simulink model "EKFsim"  (R2024b)
settings: Solver=VariableStepAuto  StartTime=0.0  StopTime=param.simul.t_end  FixedStep=1/52  RelTol=1e-3
values from neighbouring files (symbols this model uses):
  N = length(t)    [trajectory_paraglider.m]    (also in trajectory_paraglider.mat = 31201; trajectory_paraglider_backup.m; unit_test_madgwick_full_traj.m)
undefined symbols (not defined in the file or in its folder): param
libraries: nesl_utility x7, sm_lib x4
settings Model: Creator=OBWELUC  LastModifiedBy=OBWELUC
settings ExplorerConfigSet: InternalSimMechanicsExplorerSettings="<ExplorerConfiguration><canonicalview>default</canonicalview><AnimationSetting><BasePlaybackSpeed>1.0</BasePlaybackSpeed><PlaybackSpeedFactor>0.00390625</PlaybackSpeedFactor></AnimationSetting><TilePanel><TileInfo><Tiles Columns=\"2\" Count=\"4\" Rows=\"2\"><Column Weight=\"0.4997\"/><Column Weight=\"0.5003\"/><Row Weight=\"0.5\"/><Row Weight=\"0.5\"/><Tile Height=\"1\" Width=\"1\" X=\"0\" Y=\"0\"/><Tile Height=\"1\" Width=\"1\" X=\"0\" Y=\"1\"/><Tile Height=\"1\" Width=\"1\" X=\"1\" Y=\"0\"/><Tile Height=\"1\" Width=\"1\" X=\"1\" Y=\"1\"/></Tiles></TileInfo><SceneInfo><SceneViewer><BGColor><R>0.60000002384185791</R><G>0.60000002384185791</G><B>0.60000002384185791</B></BGColor><Camera><DoPerspective>off</DoPerspective><Position><X>5.29153282342771369</X><Y>-4.80631047053996685</Y><Z>2.23047224175609227</Z></Position><Center><X>1.33679013155167015</X><Y>-8.50343425895516702e-07</Y><Z>1.79372941692059129</Z></Center><Up><X>-0.00245210583782279334</X><Y>0.0884942118943543576</Y><Z>0.996073672796424003</Z></Up><ViewLimDist>1</ViewLimDist><YLim>3.61698657274246216</YLim><XLim>5.76316532752325905</XLim></Camera></SceneViewer><SceneViewer><BGColor><R>0.60000002384185791</R><G>0.60000002384185791</G><B>0.60000002384185791</B></BGColor><Camera><DoPerspective>off</DoPerspective><Position><X>2.82812637171379455</X><Y>-3.86128984680013376</Y><Z>6.51831083835967462</Z></Position><Center><X>1.10088169185850537</X><Y>-0.0853434819935348088</Y><Z>2.80557330046554076</Z></Center><Up><X>0.0701428928981585736</X><Y>0.715516230746083615</Y><Z>0.695065822864852967</Z></Up><ViewLimDist>1</ViewLimDist><YLim>5.65757834911346436</YLim><XLim>9.01456467244634929</XLim></Camera></SceneViewer><SceneViewer><BGColor><R>0.60000002384185791</R><G>0.60000002384185791</G><B>0.60000002384185791</B></BGColor><Camera><DoPerspective>off</DoPerspective><Position><X>7.61755312712227983</X><Y>-8.51291863668279802e-08</Y><Z>1.79376937141421422</Z></Position><Center><X>1.33679044539985625</X><Y>-8.51291863668279802e-08</Y><Z>1.79376937141421422</Z></Center><Up><X>-0</X><Y>0</Y><Z>1</Z></Up><ViewLimDist>1</ViewLimDist><YLim>3.61698657274246216</YLim><XLim>5.77066944904347245</XLim></Camera></SceneViewer><SceneViewer><BGColor><R>0.60000002384185791</R><G>0.60000002384185791</G><B>0.60000002384185791</B></BGColor><Camera><DoPerspective>off</DoPerspective><Position><X>4.61649383527782309</X><Y>-3.27970335927912426</Y><Z>6.03338553158868862</Z></Position><Center><X>1.39001899753018088</X><Y>-0.0532285215318148985</Y><Z>2.80691069384086322</Z></Center><Up><X>-0.408248290463863073</X><Y>0.408248290463863073</Y><Z>0.816496580927726145</Z></Up><ViewLimDist>1</ViewLimDist><YLim>4.68673889160156243</YLim><XLim>7.4773904722854807</XLim></Camera></SceneViewer></SceneInfo></TilePanel><MechEditorPanel><Cameras/><GfxPanelCameraMap/><VideoCreator><PlaybackSpeedRatio>1.0</PlaybackSpeedRatio><FrameRate>30</FrameRate><VideoFormat>Motion JPEG AVI</VideoFormat><FrameSize>auto</FrameSize></VideoCreator></MechEditorPanel></ExplorerConfiguration>"

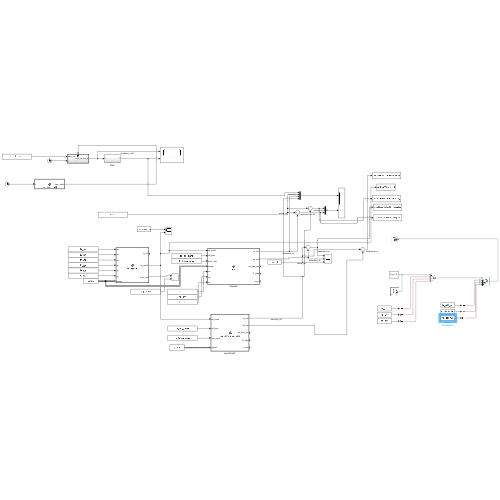
[thumbnail: Simulink's stored preview of the top-level diagram]
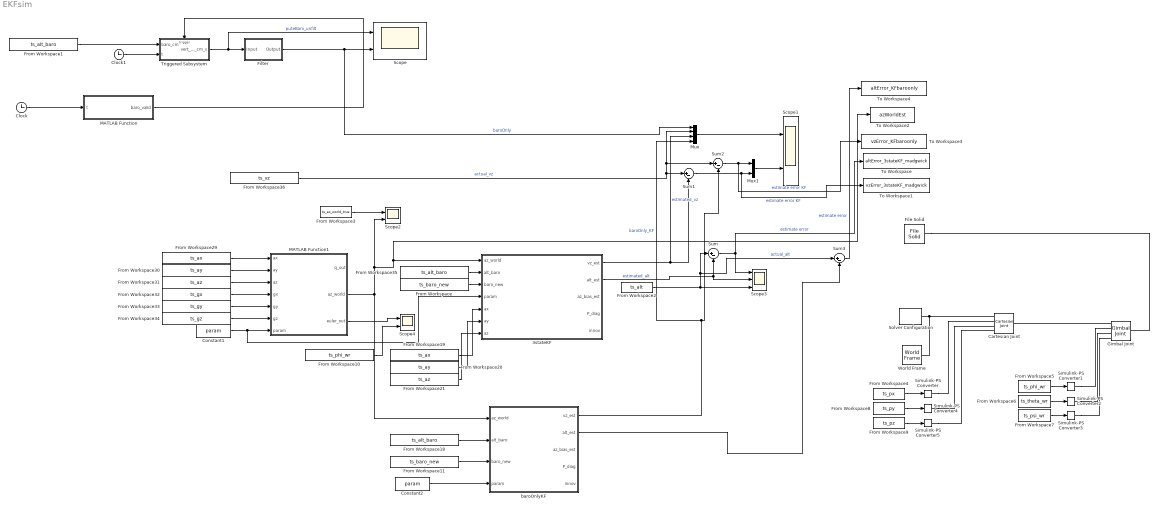
== system EKFsim ==
  3stateKF : MATLAB Function  TreatAsAtomicUnit=on  SystemSampleTime=param.dt_imu
  Cartesian Joint : sm_lib/Joints/Cartesian Joint  JointMode=Normal  CompositeWrenchDir=FollowerOnBase  CompositeWrenchFrame=BaseFrame  SenseConstraintForce=off  SenseConstraintTorque=off  SenseTotalForce=off  SenseTotalTorque=off  PxPositionTargetSpecify=off  PxPositionTargetPriority=High  PxPositionTargetValue=0  PxPositionTargetValueUnits=m  PxVelocityTargetSpecify=off  PxVelocityTargetPriority=High  PxVelocityTargetValue=0  PxVelocityTargetValueUnits=m/s  PxEquilibriumPosition=0  PxEquilibriumPositionUnits=m  PxSpringStiffness=0  PxSpringStiffnessUnits=N/m  PxDampingCoefficient=0  PxDampingCoefficientUnits=N/(m/s)  PxLowerLimitSpecify=off  PxLowerLimitBound=-1  PxLowerLimitBoundUnits=m  PxLowerLimitStiffness=1e6  PxLowerLimitStiffnessUnits=N/m  PxLowerLimitDamping=1e3  PxLowerLimitDampingUnits=N/(m/s)  PxLowerLimitTransitionRegionWidth=1e-4  PxLowerLimitTransitionRegionWidthUnits=m  PxUpperLimitSpecify=off  PxUpperLimitBound=1  PxUpperLimitBoundUnits=m  PxUpperLimitStiffness=1e6  PxUpperLimitStiffnessUnits=N/m  PxUpperLimitDamping=1e3  PxUpperLimitDampingUnits=N/(m/s)  PxUpperLimitTransitionRegionWidth=1e-4  PxUpperLimitTransitionRegionWidthUnits=m  PxTorqueActuationMode=ComputedTorque  PxMotionActuationMode=InputMotion  PxSensePosition=off  PxSenseVelocity=off  PxSenseAcceleration=off  PxSenseTorqueForce=off  PxSenseLowerLimitTorqueForce=off  PxSenseUpperLimitTorqueForce=off  PyPositionTargetSpecify=off  PyPositionTargetPriority=High  PyPositionTargetValue=0  PyPositionTargetValueUnits=m  PyVelocityTargetSpecify=off  PyVelocityTargetPriority=High  PyVelocityTargetValue=0  PyVelocityTargetValueUnits=m/s  PyEquilibriumPosition=0  PyEquilibriumPositionUnits=m  PySpringStiffness=0  PySpringStiffnessUnits=N/m  PyDampingCoefficient=0  PyDampingCoefficientUnits=N/(m/s)  PyLowerLimitSpecify=off  PyLowerLimitBound=-1  PyLowerLimitBoundUnits=m  PyLowerLimitStiffness=1e6  PyLowerLimitStiffnessUnits=N/m  PyLowerLimitDamping=1e3  PyLowerLimitDampingUnits=N/(m/s)  PyLowerLimitTransitionRegionWidth=1e-4  PyLowerLimitTransitionRegionWidthUnits=m  PyUpperLimitSpecify=off  PyUpperLimitBound=1  PyUpperLimitBoundUnits=m  PyUpperLimitStiffness=1e6  PyUpperLimitStiffnessUnits=N/m  PyUpperLimitDamping=1e3  PyUpperLimitDampingUnits=N/(m/s)  PyUpperLimitTransitionRegionWidth=1e-4  PyUpperLimitTransitionRegionWidthUnits=m  PyTorqueActuationMode=ComputedTorque  PyMotionActuationMode=InputMotion  PySensePosition=off  PySenseVelocity=off  PySenseAcceleration=off  PySenseTorqueForce=off  PySenseLowerLimitTorqueForce=off  PySenseUpperLimitTorqueForce=off  PzPositionTargetSpecify=off  PzPositionTargetPriority=High  PzPositionTargetValue=0  PzPositionTargetValueUnits=m  PzVelocityTargetSpecify=off  PzVelocityTargetPriority=High  PzVelocityTargetValue=0  PzVelocityTargetValueUnits=m/s  PzEquilibriumPosition=0  PzEquilibriumPositionUnits=m  PzSpringStiffness=0  PzSpringStiffnessUnits=N/m  PzDampingCoefficient=0  PzDampingCoefficientUnits=N/(m/s)  PzLowerLimitSpecify=off  PzLowerLimitBound=-1  PzLowerLimitBoundUnits=m  PzLowerLimitStiffness=1e6  PzLowerLimitStiffnessUnits=N/m  PzLowerLimitDamping=1e3  PzLowerLimitDampingUnits=N/(m/s)  PzLowerLimitTransitionRegionWidth=1e-4  PzLowerLimitTransitionRegionWidthUnits=m  PzUpperLimitSpecify=off  PzUpperLimitBound=1  PzUpperLimitBoundUnits=m  PzUpperLimitStiffness=1e6  PzUpperLimitStiffnessUnits=N/m  PzUpperLimitDamping=1e3  PzUpperLimitDampingUnits=N/(m/s)  PzUpperLimitTransitionRegionWidth=1e-4  PzUpperLimitTransitionRegionWidthUnits=m  PzTorqueActuationMode=ComputedTorque  PzMotionActuationMode=InputMotion  PzSensePosition=off  PzSenseVelocity=off  PzSenseAcceleration=off  PzSenseTorqueForce=off  PzSenseLowerLimitTorqueForce=off  PzSenseUpperLimitTorqueForce=off
  Clock : Clock
  Clock1 : Clock
  Constant1 : Constant  Value=param  OutDataTypeStr=Bus: BusKF
  Constant2 : Constant  Value=param  OutDataTypeStr=Bus: BusKF
  File Solid : sm_lib/Body Elements/File Solid  ExtGeomFileName=C:\Users\OBWELUC\Desktop\miniVarioCode\kf\Assemblage paramoteur.STEP  UnitType=FromFile  ExtGeomFileUnits=m  StepReaderType=HEX  ExportConvexHullGeometry=off  InertiaType=PointMass  BasedOnType=DensityFromFile  Density=1000  DensityUnits=kg/m^3  Mass=1  MassUnits=kg  CenterOfMass=[0 0 0]  CenterOfMassUnits=m  MomentsOfInertia=[1 1 1]  MomentsOfInertiaUnits=kg*m^2  ProductsOfInertia=[0 0 0]  ProductsOfInertiaUnits=kg*m^2  GraphicType=FromGeometry  MarkerShape=Sphere  MarkerSize=10  GraphicVisPropType=SimpleVisualProperties  GraphicDiffuseColor=[0.5 0.5 0.5]  GraphicOpacity=1  GraphicSpecularColor=[0.5 0.5 0.5 1.0]  GraphicAmbientColor=[0.15 0.15 0.15 1.0]  GraphicEmissiveColor=[0.0 0.0 0.0 1.0]  GraphicShininess=75  DoExposeReferenceFrame=off  SerializedFrames=<Frames><Frame><Id>Frame1</Id><Value><Name>Fcorr</Name><Origin><Source>ReferenceFrame</Source><FeatureName></FeatureName></Origin><PrimaryAxis><DefinedDirection>+X</DefinedDirection><Source>ReferenceFrame</Source><SourceDirection>+Z</SourceDirection><FeatureName></FeatureName></PrimaryAxis><SecondaryAxis><DefinedDirection>+Y</DefinedDirection><Source>ReferenceFrame</Source><SourceDirection>+X</SourceDirection><FeatureName></FeatureName></SecondaryAxis></Value></Frame></Frames>
  Filter : Subsystem  Tag=FilterWizardSubSystem
      settings: ErrorFcn=dspFilterRealizedInBasicElemsAlgLoopErrFcnCallback
  From Workspace : FromWorkspace  VariableName=ts_baro_new  SampleTime=param.dt_imu
  From Workspace1 : FromWorkspace  VariableName=ts_alt_baro  SampleTime=1/52
  From Workspace10 : FromWorkspace  VariableName=ts_phi_wr  SampleTime=param.dt_imu
  From Workspace11 : FromWorkspace  VariableName=ts_baro_new  SampleTime=param.dt_imu
  From Workspace18 : FromWorkspace  VariableName=ts_alt_baro  SampleTime=param.dt_imu
  From Workspace19 : FromWorkspace  VariableName=ts_ax  SampleTime=param.dt_imu
  From Workspace2 : FromWorkspace  VariableName=ts_alt  SampleTime=1/52
  From Workspace20 : FromWorkspace  VariableName=ts_ay  SampleTime=param.dt_imu
  From Workspace21 : FromWorkspace  VariableName=ts_az  SampleTime=param.dt_imu
  From Workspace29 : FromWorkspace  VariableName=ts_ax  SampleTime=param.dt_imu
  From Workspace3 : FromWorkspace  VariableName=ts_az_world_true
  From Workspace30 : FromWorkspace  VariableName=ts_ay  SampleTime=param.dt_imu
  From Workspace31 : FromWorkspace  VariableName=ts_az  SampleTime=param.dt_imu
  From Workspace32 : FromWorkspace  VariableName=ts_gx  SampleTime=param.dt_imu
  From Workspace33 : FromWorkspace  VariableName=ts_gy  SampleTime=param.dt_imu
  From Workspace34 : FromWorkspace  VariableName=ts_gz  SampleTime=param.dt_imu
  From Workspace35 : FromWorkspace  VariableName=ts_alt_baro  SampleTime=param.dt_imu
  From Workspace36 : FromWorkspace  VariableName=ts_vz  SampleTime=1/52
  From Workspace4 : FromWorkspace  VariableName=ts_px  SampleTime=-1
  From Workspace5 : FromWorkspace  VariableName=ts_phi_wr  SampleTime=-1
  From Workspace6 : FromWorkspace  VariableName=ts_theta_wr  SampleTime=-1
  From Workspace7 : FromWorkspace  VariableName=ts_psi_wr  SampleTime=-1
  From Workspace8 : FromWorkspace  VariableName=ts_py  SampleTime=-1
  From Workspace9 : FromWorkspace  VariableName=ts_pz  SampleTime=-1
  Gimbal Joint : sm_lib/Joints/Gimbal Joint  JointMode=Normal  CompositeWrenchDir=FollowerOnBase  CompositeWrenchFrame=BaseFrame  SenseConstraintForce=off  SenseConstraintTorque=off  SenseTotalForce=off  SenseTotalTorque=off  RxPositionTargetSpecify=off  RxPositionTargetPriority=High  RxPositionTargetValue=0  RxPositionTargetValueUnits=deg  RxVelocityTargetSpecify=off  RxVelocityTargetPriority=High  RxVelocityTargetValue=0  RxVelocityTargetValueUnits=deg/s  RxEquilibriumPosition=0  RxEquilibriumPositionUnits=deg  RxSpringStiffness=0  RxSpringStiffnessUnits=N*m/deg  RxDampingCoefficient=0  RxDampingCoefficientUnits=N*m/(deg/s)  RxLowerLimitSpecify=off  RxLowerLimitBound=-90  RxLowerLimitBoundUnits=deg  RxLowerLimitStiffness=1e4  RxLowerLimitStiffnessUnits=N*m/deg  RxLowerLimitDamping=10  RxLowerLimitDampingUnits=N*m/(deg/s)  RxLowerLimitTransitionRegionWidth=0.1  RxLowerLimitTransitionRegionWidthUnits=deg  RxUpperLimitSpecify=off  RxUpperLimitBound=90  RxUpperLimitBoundUnits=deg  RxUpperLimitStiffness=1e4  RxUpperLimitStiffnessUnits=N*m/deg  RxUpperLimitDamping=10  RxUpperLimitDampingUnits=N*m/(deg/s)  RxUpperLimitTransitionRegionWidth=0.1  RxUpperLimitTransitionRegionWidthUnits=deg  RxTorqueActuationMode=ComputedTorque  RxMotionActuationMode=InputMotion  RxSensePosition=off  RxSenseVelocity=off  RxSenseAcceleration=off  RxSenseTorqueForce=off  RxSenseLowerLimitTorqueForce=off  RxSenseUpperLimitTorqueForce=off  RyPositionTargetSpecify=off  RyPositionTargetPriority=High  RyPositionTargetValue=0  RyPositionTargetValueUnits=deg  RyVelocityTargetSpecify=off  RyVelocityTargetPriority=High  RyVelocityTargetValue=0  RyVelocityTargetValueUnits=deg/s  RyEquilibriumPosition=0  RyEquilibriumPositionUnits=deg  RySpringStiffness=0  RySpringStiffnessUnits=N*m/deg  RyDampingCoefficient=0  RyDampingCoefficientUnits=N*m/(deg/s)  RyLowerLimitSpecify=off  RyLowerLimitBound=-90  RyLowerLimitBoundUnits=deg  RyLowerLimitStiffness=1e4  RyLowerLimitStiffnessUnits=N*m/deg  RyLowerLimitDamping=10  RyLowerLimitDampingUnits=N*m/(deg/s)  RyLowerLimitTransitionRegionWidth=0.1  RyLowerLimitTransitionRegionWidthUnits=deg  RyUpperLimitSpecify=off  RyUpperLimitBound=90  RyUpperLimitBoundUnits=deg  RyUpperLimitStiffness=1e4  RyUpperLimitStiffnessUnits=N*m/deg  RyUpperLimitDamping=10  RyUpperLimitDampingUnits=N*m/(deg/s)  RyUpperLimitTransitionRegionWidth=0.1  RyUpperLimitTransitionRegionWidthUnits=deg  RyTorqueActuationMode=ComputedTorque  RyMotionActuationMode=InputMotion  RySensePosition=off  RySenseVelocity=off  RySenseAcceleration=off  RySenseTorqueForce=off  RySenseLowerLimitTorqueForce=off  RySenseUpperLimitTorqueForce=off  RzPositionTargetSpecify=off  RzPositionTargetPriority=High  RzPositionTargetValue=0  RzPositionTargetValueUnits=deg  RzVelocityTargetSpecify=off  RzVelocityTargetPriority=High  RzVelocityTargetValue=0  RzVelocityTargetValueUnits=deg/s  RzEquilibriumPosition=0  RzEquilibriumPositionUnits=deg  RzSpringStiffness=0  RzSpringStiffnessUnits=N*m/deg  RzDampingCoefficient=0  RzDampingCoefficientUnits=N*m/(deg/s)  RzLowerLimitSpecify=off  RzLowerLimitBound=-90  RzLowerLimitBoundUnits=deg  RzLowerLimitStiffness=1e4  RzLowerLimitStiffnessUnits=N*m/deg  RzLowerLimitDamping=10  RzLowerLimitDampingUnits=N*m/(deg/s)  RzLowerLimitTransitionRegionWidth=0.1  RzLowerLimitTransitionRegionWidthUnits=deg  RzUpperLimitSpecify=off  RzUpperLimitBound=90  RzUpperLimitBoundUnits=deg  RzUpperLimitStiffness=1e4  RzUpperLimitStiffnessUnits=N*m/deg  RzUpperLimitDamping=10  RzUpperLimitDampingUnits=N*m/(deg/s)  RzUpperLimitTransitionRegionWidth=0.1  RzUpperLimitTransitionRegionWidthUnits=deg  RzTorqueActuationMode=ComputedTorque  RzMotionActuationMode=InputMotion  RzSensePosition=off  RzSenseVelocity=off  RzSenseAcceleration=off  RzSenseTorqueForce=off  RzSenseLowerLimitTorqueForce=off  RzSenseUpperLimitTorqueForce=off
  MATLAB Function : MATLAB Function  TreatAsAtomicUnit=on
  MATLAB Function1 : MATLAB Function  TreatAsAtomicUnit=on  SystemSampleTime=param.dt_imu
  Mux : Mux
  Mux1 : Mux  Inputs=2
  Scope{,1..2,4} (4 alike) : Scope  NumInputPorts=2
  Scope3 : Scope  NumInputPorts=3
  Simulink-PS Converter{,1..5} (6 alike) : nesl_utility/Simulink-PS Converter  PhysicalDomain=network_engine_domain  SubClassName=ps_input  LeftPortType=input  RightPortType=output  PseudoPeriodic=off  Frequencies=[]  NoiseDistribution=none  NoiseParameters=[]  Unit=1  AffineConversion=off  FilteringAndDerivatives=filter  SimscapeFilterOrder=2  InputFilterTimeConstant=0.001  UdotUserProvided=0
  Solver Configuration : nesl_utility/Solver Configuration  PhysicalDomain=network_engine_domain  SubClassName=solver  LeftPortType=input  RightPortType=generic  Tones=[]  Harmonics=[]  SimulateNoise=off  Profile=off  UseLocalSampling=off  EnableSwitchedLinearOptims=on  FrequencyDomain=off  UseCCode=off  RelTol=0.001  AbsTol=0.001  MinStep=1e-09  ToWorkspace=off  RevertToSquareIcSolve=off  NumHomotopyIterations=100  PhasorMode=off  PhasorModeNumHarmonics=1  ConsistencySolver=NEWTON_XTOL_AFTER_FTOL  IndexReductionMethod=DerivativeReplacement  DoDC=off  ResidualTolerance=1e-09  ConsistencyTolSource=GLOBAL  ConsistencyAbsTol=0.001  ConsistencyRelTol=0.001  ConsistencyTolFactor=0.001  UseLocalSolver=off  LocalSolverChoice=NE_BACKWARD_EULER_ADVANCER  ResolveIndetEquations=on  FunctionEvalNumThread=1  LocalSolverSampleTime=0.001  DoFixedCost=off  MaxNonlinIter=3  MaxModeIter=2  ComputeImpulses=off  ImpulseIterations=2  LinearAlgebra=auto  LinearAlgebraNumThread=0  EquationFormulation=NE_TIME_EF  DelaysMemoryBudget=1024  AutomaticFiltering=on  FilteringTimeConstant=0.001  PartitionStorageMethod=AS_NEEDED  PartitionMemoryBudget=1024  PartitionMethod=ROBUST  MultibodyUseLocalSolver=off  MultibodyLocalSolverChoice=ODE1  MultibodyLocalSolverSampleTime=0.001
  Sum{,1..3} (4 alike) : Sum  Inputs=|+-
  To Workspace : ToWorkspace  VariableName=altError_3stateKF_madgwick  SaveFormat=Timeseries  SampleTime=-1
  To Workspace1 : ToWorkspace  VariableName=vzError_3stateKF_madgwick  SaveFormat=Timeseries  SampleTime=-1
  To Workspace2 : ToWorkspace  VariableName=azWorldEst  SaveFormat=Timeseries  SampleTime=-1
  To Workspace3 : ToWorkspace  VariableName=vzError_KFbaroonly  SaveFormat=Timeseries  SampleTime=-1
  To Workspace4 : ToWorkspace  VariableName=altError_KFbaroonly  SaveFormat=Timeseries  SampleTime=-1
  Triggered Subsystem : Subsystem  TreatAsAtomicUnit=on
  World Frame : sm_lib/Frames and Transforms/World Frame
  baroOnlyKF : MATLAB Function  TreatAsAtomicUnit=on
  wires:
  MATLAB Function/1(baro_valid) -> Triggered Subsystem/Trigger
  Clock/1 -> MATLAB Function/1(t)
  Clock1/1 -> Triggered Subsystem/2(t)
  Triggered Subsystem/1(vert_vel_cm_s) -> Scope/1, Filter/1(Input)  "puteBaro_unfilt"
  Constant1/1 -> 3stateKF/4(param), MATLAB Function1/7(param)
  From Workspace29/1 -> MATLAB Function1/1(ax)
  From Workspace30/1 -> MATLAB Function1/2(ay)
  From Workspace31/1 -> MATLAB Function1/3(az)
  From Workspace32/1 -> MATLAB Function1/4(gx)
  From Workspace33/1 -> MATLAB Function1/5(gy)
  From Workspace34/1 -> MATLAB Function1/6(gz)
  MATLAB Function1/2(az_world) -> baroOnlyKF/1(az_world), 3stateKF/1(az_world), To Workspace2/1, Scope2/2
  From Workspace35/1 -> 3stateKF/2(alt_baro)
  From Workspace1/1 -> Triggered Subsystem/1(baro_cm)
  From Workspace/1 -> 3stateKF/3(baro_new)
  From Workspace4/1 -> Simulink-PS Converter/1
  From Workspace5/1 -> Simulink-PS Converter1/1
  From Workspace7/1 -> Simulink-PS Converter3/1
  From Workspace6/1 -> Simulink-PS Converter2/1
  From Workspace8/1 -> Simulink-PS Converter4/1
  From Workspace9/1 -> Simulink-PS Converter5/1
  3stateKF/2(alt_est) -> Scope3/2, Sum/2  "estimated_alt"
  From Workspace2/1 -> Sum3/1, Sum/1, Scope3/3  "actual_alt"
  Sum/1 -> Scope3/1, To Workspace/1  "estimate error"
  3stateKF/1(vz_est) -> Sum1/2, Mux/3  "estimated_vz"
  From Workspace36/1 -> Sum1/1, Sum2/1, Mux/2  "actual_vz"
  Filter/1(Output) -> Mux/1, Scope/2  "baroOnly"
  Mux/1 -> Scope1/1
  Mux1/1 -> Scope1/2
  Sum1/1 -> To Workspace1/1, Mux1/2  "estimate error KF"
  Sum2/1 -> To Workspace3/1, Mux1/1  "estimate error KF"
  From Workspace11/1 -> baroOnlyKF/3(baro_new)
  From Workspace18/1 -> baroOnlyKF/2(alt_baro)
  Constant2/1 -> baroOnlyKF/4(param)
  From Workspace19/1 -> 3stateKF/5(ax)
  From Workspace20/1 -> 3stateKF/6(ay)
  From Workspace21/1 -> 3stateKF/7(az)
  baroOnlyKF/1(vz_est) -> Mux/4, Sum2/2  "baroOnly_KF"
  From Workspace3/1 -> Scope2/1
  MATLAB Function1/3(euler_out) -> Scope4/1
  From Workspace10/1 -> Scope4/2
  baroOnlyKF/2(alt_est) -> Sum3/2
  Sum3/1 -> To Workspace4/1  "estimate error"
  connections:
  Solver Configuration/RConn1 -- Cartesian Joint/LConn1 -- World Frame/RConn1
  File Solid/LConn1 -- Gimbal Joint/RConn1
  Gimbal Joint/LConn1 -- Cartesian Joint/RConn1
  Simulink-PS Converter/RConn1 -- Cartesian Joint/LConn2
  Simulink-PS Converter2/RConn1 -- Gimbal Joint/LConn3
  Simulink-PS Converter1/RConn1 -- Gimbal Joint/LConn2
  Simulink-PS Converter3/RConn1 -- Gimbal Joint/LConn4
  Simulink-PS Converter4/RConn1 -- Cartesian Joint/LConn3
  Simulink-PS Converter5/RConn1 -- Cartesian Joint/LConn4

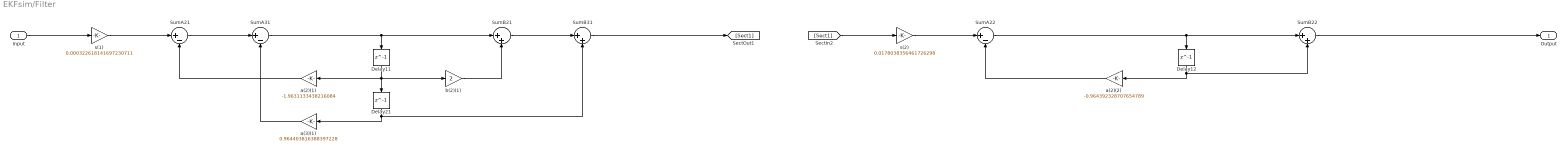
== system EKFsim/Filter ==
  Input : Inport
  Delay11 : Delay  DelayLength=1  InitialCondition=0
  Delay12 : Delay  DelayLength=1  InitialCondition=0
  Delay21 : Delay  DelayLength=1  InitialCondition=0
  SumA21 : Sum  Inputs=|+-  RndMeth=Nearest  SaturateOnIntegerOverflow=on  OutDataTypeStr=Inherit: Same as first input
  SumA22 : Sum  Inputs=|+-  RndMeth=Nearest  SaturateOnIntegerOverflow=on  OutDataTypeStr=Inherit: Same as first input
  SumA31 : Sum  Inputs=|+-  RndMeth=Nearest  SaturateOnIntegerOverflow=on  OutDataTypeStr=Inherit: Same as first input
  SumB21 : Sum  Inputs=|++  RndMeth=Nearest  SaturateOnIntegerOverflow=on  OutDataTypeStr=Inherit: Same as first input
  SumB22 : Sum  Inputs=|++  RndMeth=Nearest  SaturateOnIntegerOverflow=on  OutDataTypeStr=Inherit: Same as first input
  SumB31 : Sum  Inputs=|++  RndMeth=Nearest  SaturateOnIntegerOverflow=on  OutDataTypeStr=Inherit: Same as first input
  a(2)(1) : Gain  Gain=-1.9631133438216084  ParamDataTypeStr=double  RndMeth=Nearest  SaturateOnIntegerOverflow=on  OutDataTypeStr=Inherit: Same as input
  a(2)(2) : Gain  Gain=-0.964392328707654789  ParamDataTypeStr=double  RndMeth=Nearest  SaturateOnIntegerOverflow=on  OutDataTypeStr=Inherit: Same as input
  a(3)(1) : Gain  Gain=0.964403816388397228  ParamDataTypeStr=double  RndMeth=Nearest  SaturateOnIntegerOverflow=on  OutDataTypeStr=Inherit: Same as input
  b(2)(1) : Gain  Gain=2  ParamDataTypeStr=double  RndMeth=Nearest  SaturateOnIntegerOverflow=on  OutDataTypeStr=Inherit: Same as input
  s(1) : Gain  Gain=0.000322618141697230711  ParamDataTypeStr=double  RndMeth=Nearest  SaturateOnIntegerOverflow=on  OutDataTypeStr=Inherit: Same as input
  s(2) : Gain  Gain=0.0178038356461726298  ParamDataTypeStr=double  RndMeth=Nearest  SaturateOnIntegerOverflow=on  OutDataTypeStr=Inherit: Same as input
  Output : Outport
  wires:
  Input/1 -> s(1)/1
  s(1)/1 -> SumA21/1
  SumA21/1 -> SumA31/1
  SumA31/1 -> SumB21/1, Delay11/1
  SumB21/1 -> SumB31/1
  SumB31/1 -> [Sect1]
  a(2)(1)/1 -> SumA21/2
  Delay11/1 -> a(2)(1)/1, b(2)(1)/1, Delay21/1
  b(2)(1)/1 -> SumB21/2
  a(3)(1)/1 -> SumA31/2
  Delay21/1 -> a(3)(1)/1, SumB31/2
  [Sect1] -> s(2)/1
  s(2)/1 -> SumA22/1
  SumA22/1 -> SumB22/1, Delay12/1
  SumB22/1 -> Output/1
  a(2)(2)/1 -> SumA22/2
  Delay12/1 -> a(2)(2)/1, SumB22/2

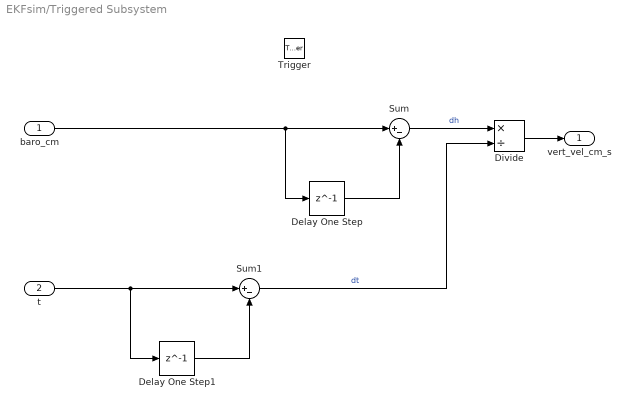
== system EKFsim/Triggered Subsystem ==
  baro_cm : Inport
  t : Inport  Port=2
  Trigger : TriggerPort  VariantControl=(inherit)
  Delay One Step : Delay  DelayLength=1
  Delay One Step1 : Delay  DelayLength=1
  Divide : Product  Inputs=*/
  Sum : Sum  Inputs=|+-
  Sum1 : Sum  Inputs=|+-
  vert_vel_cm_s : Outport
  wires:
  baro_cm/1 -> Sum/1, Delay One Step/1
  Delay One Step/1 -> Sum/2
  Sum/1 -> Divide/1  "dh"
  t/1 -> Delay One Step1/1, Sum1/1
  Delay One Step1/1 -> Sum1/2
  Sum1/1 -> Divide/2  "dt"
  Divide/1 -> vert_vel_cm_s/1

== matlab function EKFsim/MATLAB Function ==
  data: t input; baro_valid output
function baro_valid = gen_baro_valid(t)
  baro_valid = mod(round(t * 52), 7) == 0;
end

== matlab function EKFsim/3stateKF ==
  data: az_world input; vz_est output; alt_baro input; baro_new input; param input Bus: BusKF; alt_est output; az_bias_est output; P_diag output; innov output; ax input; ay input; az input
function [vz_est, alt_est, az_bias_est, P_diag, innov] = ...
         KF(az_world, alt_baro, baro_new, param, ax, ay, az)
    [vz_est, alt_est, az_bias_est, P_diag, innov] = fcn_kalman_vz(az_world, alt_baro, baro_new, param, ax, ay, az);
end

== matlab function EKFsim/MATLAB Function1 ==
  data: ax input; q_out output; ay input; az input; gx input; gy input; gz input; param input Bus: BusKF; az_world output; euler_out output
function [q_out, az_world, euler_out] = madgwick(ax, ay, az, gx, gy, gz, param)
    [q_out, az_world, euler_out] = fcn_madgwick(ax, ay, az, gx, gy, gz, param);
end

== matlab function EKFsim/baroOnlyKF ==
  data: az_world input; vz_est output; alt_baro input; baro_new input; param input Bus: BusKF; alt_est output; az_bias_est output; P_diag output; innov output
function [vz_est, alt_est, az_bias_est, P_diag, innov] = ...
         fcn_kalman_vz_baro(az_world, alt_baro, baro_new, param)
%FCN_KALMAN_VZ_BARO  Baro-primary Kalman filter for vertical speed estimation.
%
%  Architecture: barometer is the PRIMARY sensor and drives all meaningful
%  state corrections. The IMU (az_world from Madgwick) is used ONLY as a
%  predictor between baro samples — its contribution is heavily discounted
%  so that attitude errors during banked thermals do not corrupt the estimate.
%
%  Motivation: during banked turns (45°–55°), Madgwick's az_world contains
%  systematic tilt errors that are larger than the baro noise. Letting the
%  KF trust the IMU in those conditions actively worsens vz accuracy.
%  By setting u=0 (zero-acceleration prediction) and inflating Q to cover
%  the real vz dynamics, the baro update at 8 Hz carries the estimate and
%  the IMU error is absorbed into the process noise.
%
% =========================================================================
%  STATE VECTOR   x = [h; vz; az_bias]
%    h        : altitude above reference [m], up positive
%    vz       : vertical speed [m/s], up positive
%    az_bias  : residual vertical accel bias [m/s²] — kept for interface
%               compatibility; with u=0 it absorbs mean IMU offset.
%
%  INPUTS
%    az_world  : Madgwick world-frame vertical specific force [m/s²]
%                Used only when IMU blending is enabled (see IMU_BLEND_WEIGHT).
%                Set IMU_BLEND_WEIGHT=0 to ignore entirely.
%    alt_baro  : barometer altitude measurement [m]  (ZOH from 8 Hz)
%    baro_new  : flag — 1 = new baro sample this step, 0 = old
%    param     : parameter bus (param_init.m)
%
%  OUTPUTS  (identical interface to fcn_kalman_vz.m for drop-in replacement)
%    vz_est      : estimated vertical speed [m/s], up positive
%    alt_est     : estimated altitude [m]
%    az_bias_est : estimated accel bias [m/s²]
%    P_diag      : diagonal of P (3×1)
%    innov       : baro innovation [m]  (NaN when no new measurement)
%
%  KEY DESIGN CHOICES vs fcn_kalman_vz.m
%  -----------------------------------------------------------------------
%  1. Control input u = IMU_BLEND_WEIGHT * (-(az_world+g))
%     Default IMU_BLEND_WEIGHT = 0  →  zero-input prediction.
%     The predictor becomes: h_{k+1} = h_k + dt*vz_k
%                            vz_{k+1} = vz_k
%     vz is held constant between baro updates, which is correct on average
%     for a variometer (vz changes slowly relative to baro rate).
%
%  2. Q is set independently of param.kf.Q.
%     Q must be large enough that P grows sufficiently between baro updates
%     so the baro gain K is meaningful (~0.5–0.9 on the h channel).
%     Q_vz drives how quickly the filter can track vz changes.
%     Rule of thumb: sqrt(Q_vz * dt_baro) ≈ expected vz change per baro step.
%     At 8 Hz, a thermal onset can change vz by ~0.5 m/s in 0.125 s →
%     Q_vz ≈ (0.5/0.125)^2 * dt_imu ≈ 16 * (1/52) ≈ 0.31 m/s² per root-Hz.
%     We use a slightly more conservative value tunable via Q_VZ_SIGMA below.
%
%  3. Baro update uses the same R as param.kf.R_h (tunable separately).
%     The innovation gate is retained for outlier rejection.
%
%  SIMULINK USAGE
%    Drop-in replacement for fcn_kalman_vz.m.
%    Same port order, same sample time (param.dt_imu).
%    az_world input can be left connected — it is weighted to zero by default.
%
%#codegen

%% =========================================================
%  TUNING CONSTANTS  (edit here, not in param_init for now)
% ==========================================================

% Weight on IMU control input [0 = baro-only, 1 = full IMU trust]
% Set to 0 for pure baro-primary. Set to 0.1–0.3 to blend lightly.
IMU_BLEND_WEIGHT = 0;

% Process noise for vz [m/s per sqrt(Hz)]
% Governs how fast the filter tracks vz changes between baro updates.
% Increase if vz RMSE is large during rapid thermal entries.
% Decrease if the estimate is noisy during stable glide.
% Suggested range: 0.1 – 0.5
Q_VZ_SIGMA = 0.5;   % [m/s / sqrt(Hz)]

% Process noise for altitude [m per sqrt(Hz)]
% Usually much smaller than vz — altitude is the integrated state.
Q_H_SIGMA  = 0.01;  % [m / sqrt(Hz)]

% Process noise for bias [m/s² per sqrt(Hz)]
% With u=0, the bias state absorbs the mean IMU offset.
% Keep small so it doesn't destabilise; it's largely irrelevant here.
Q_BIAS_SIGMA = 0.005;  % [m/s² / sqrt(Hz)]

%% =========================================================
%  PERSISTENT STATE
% ==========================================================
persistent x_est P initialised;

if isempty(initialised)
    x_est      = param.kf.x0(:);
    x_est(1)   = alt_baro;        % warm-start altitude from first baro reading
    P          = param.kf.P0;
    initialised = true;
end

%% =========================================================
%  SYSTEM MATRICES
% ==========================================================
g    = param.simul.g;
dt   = param.dt_imu;

% State transition — identical to original (kinematics are exact)
%   h_{k+1}  = h_k + dt*vz_k - dt²/2 * az_bias_k   (bias correction term)
%   vz_{k+1} = vz_k           - dt   * az_bias_k
%   bias_{k+1} = bias_k
% With u=0, the -dt²/2*bias and -dt*bias terms are the only IMU influence.
F = param.kf.F;    % [1 dt -dt²/2; 0 1 -dt; 0 0 1]
B = param.kf.B;    % [dt²/2; dt; 0]
H = param.kf.H;    % [1 0 0]
R = param.kf.R_h;
gate = param.kf.gate_threshold;

% Build Q from sigma values above (continuous → discrete)
Q = diag([ Q_H_SIGMA^2  * dt, ...
           Q_VZ_SIGMA^2 * dt, ...
           Q_BIAS_SIGMA^2 * dt ]);

%% =========================================================
%  CONTROL INPUT
%  u = 0 by default (baro-primary mode).
%  With IMU_BLEND_WEIGHT > 0, lightly mix the IMU-derived acceleration.
% ==========================================================
u_imu = -(az_world + g);   % IMU vertical accel, up positive [m/s²]
u     = IMU_BLEND_WEIGHT * u_imu;
% Bias is still subtracted implicitly via F*x (x(3) = az_bias).
% With u=0, F*x propagates: h += dt*vz - dt²/2*bias, vz -= dt*bias.
% Since bias is estimated near zero (no IMU driving it), this effectively
% gives h_{k+1} ≈ h_k + dt*vz_k and vz_{k+1} ≈ vz_k.

%% =========================================================
%  PREDICTION STEP
% ==========================================================
x_pred = F * x_est + B * u;
P_pred = F * P * F' + Q;
P_pred = 0.5 * (P_pred + P_pred');   % symmetrise

%% =========================================================
%  UPDATE STEP  (only on new baro sample)
% ==========================================================
innov = NaN;

if baro_new >= 0.5
    y = alt_baro - H * x_pred;     % innovation [m]
    S = H * P_pred * H' + R;       % innovation covariance (scalar)

    % Chi-squared gate — reject outliers (|y| > ~3.3*sigma_h)
    if (y^2 / S) <= gate
        K      = P_pred * H' / S;           % Kalman gain [3×1]
        x_pred = x_pred + K * y;

        % Joseph-form covariance update (numerically stable)
        I_KH   = eye(3) - K * H;
        P_pred = I_KH * P_pred * I_KH' + K * R * K';
        P_pred = 0.5 * (P_pred + P_pred');

        innov  = y;
    end
end

%% =========================================================
%  STORE & CLIP
% ==========================================================
x_est = x_pred;
P     = P_pred;

% Physical floor — can't go underground
if x_est(1) < 0
    x_est(1) = 0;
    if x_est(2) < 0
        x_est(2) = 0;
    end
end

% Bias clip — with u=0 this should stay near zero anyway
x_est(3) = max(-2.0, min(2.0, x_est(3)));

%% =========================================================
%  OUTPUTS
% ==========================================================
vz_est      = x_est(2);
alt_est     = x_est(1);
az_bias_est = x_est(3);
P_diag      = diag(P);

end  % fcn_kalman_vz_baro
